simulink model "dVRK_RDOBS"  (Simulink 8.5)
settings: Solver=ode4  StartTime=0.0  StopTime=length(Tm)/1000  FixedStep=0.001  RelTol=1e-3
libraries: neural x630
(part 8 of 14)

== system dVRK_RDOBS/Joint 3 NN Dyn Ident/Layer 2/Delays 1 ==
  "p{2}" : Inport  PortDimensions=100  SampleTime=0.001
      mask Display: e = 0.06;c1 = [120 230 180]/255;c2 = ([120 230 180]+0)/(256+128);c3 = ([120 230 180]+128)/(256+128);patch([0 1 1 0],[0 0 1 1],c1);patch([0 1 1 1-e 1-e 0+e],[0 0 1 1-e 0+e 0+e],c2);patch([0 0 1 1-e 0+e 0+e],[0 1 1 1-e 1-e 0+e],c3);plot([0 1 1 0 0],[0 0 1 1 0]);
  mux : Mux  Inputs=1
      mask Display: e = 0.06;c1 = [120 150 230]/255;c2 = ([120 150 230]+0)/383;c3 = ([120 150 230]+128)/383;patch([0 1 1 0],[0 0 1 1],c1);patch([0 1 1 1-e 1-e 0+e],[0 0 1 1-e 0+e 0+e],c2);patch([0 0 1 1-e 0+e 0+e],[0 1 1 1-e 1-e 0+e],c3);plot([0 1 1 0 0],[0 0 1 1 0]);disp('Mux')
  "pd{2,1}" : Outport
      mask Display: e = 0.06;c1 = [120 230 180]/255;c2 = ([120 230 180]+0)/(256+128);c3 = ([120 230 180]+128)/(256+128);patch([0 1 1 0],[0 0 1 1],c1);patch([0 1 1 1-e 1-e 0+e],[0 0 1 1-e 0+e 0+e],c2);patch([0 0 1 1-e 0+e 0+e],[0 1 1 1-e 1-e 0+e],c3);plot([0 1 1 0 0],[0 0 1 1 0]);
  wires:
  "p{2}"/1 -> mux/1
  mux/1 -> "pd{2,1}"/1

== system dVRK_RDOBS/Joint 3 NN Dyn Ident/Layer 2/LW{2,1} ==
  "ad{2,1}" : Inport  PortDimensions=100  SampleTime=0.001
      mask Display: e = 0.06;c1 = [120 230 180]/255;c2 = ([120 230 180]+0)/(256+128);c3 = ([120 230 180]+128)/(256+128);patch([0 1 1 0],[0 0 1 1],c1);patch([0 1 1 1-e 1-e 0+e],[0 0 1 1-e 0+e 0+e],c2);patch([0 0 1 1-e 0+e 0+e],[0 1 1 1-e 1-e 0+e],c3);plot([0 1 1 0 0],[0 0 1 1 0]);
  "IW{2,1}(1,:)'" : Constant  Value=[-5.167254955505955;-1.8178436445965449;0.49211737404768147;-9.6830838662498326;-0.46755168693201082;1.7607856309859413;-0.084806969807460483;-1.5622860912871561;7.5100372282854364;-2.1948916538943264;0.1912546475987992;-3.4270018672278848;-7.3623865629808263;0.19766346350380701;0.48730997980870927;-0.20506493745529994;0.97745193864204638;0.16679036054209562;-0.17884970513459647;1.9736899383298294;-5.4772991886942579;-1.790933673981175;-3.5080464351406011;5.9822819492171488;2.8364180748438179;-0.2988913579922941;-0.072856020157372761;0.50318968999564839;2.3004396982929927;-0.15251543459787451;0.38654204560049144;-0.12940943559812457;2.832022145217802;-0.079145330621644708;-3.665648676122002;0.64287255965203383;3.931764786546037;-14.695817579739888;1.7362168126307793;0.36258126436183791;-1.9217057854420962;-0.29141146109069621;0.36160509862601681;0.76797790034887881;-1.7367991317149585;0.24018980699277243;-0.17825727249647286;-8.5366323143553746;0.13345769845967898;0.074840121060482059;1.4133773384275701;7.2423394399605971;0.070864353182638604;-0.10274757387060757;6.6363585532346834;0.60239026014106689;0.80956917570838027;0.62488754158380544;-0.17406692748002811;0.14812230476266114;-0.060128694573264654;0.56295323019274213;3.6621750916124358;-0.089541099264920349;-4.7357752009613723;0.19395813900816228;0.39853932795452873;0.14586909711395502;2.8018510438589299;-0.13038626499226821;0.50273892591220448;-0.17133267817527792;-0.22954196155175274;-0.54269745136298531;0.065188835392689465;-2.2926499451203948;0.3048007042901813;0.10233878512655985;0.42283871492618447;8.6505700551897551;-0.78592801250530531;12.737499354908245;0.47870971246031363;0.067869173127585336;0.14627490753962932;9.5380427871377513;0.32047634259962282;-0.056075778679940104;-0.09930934114651277;-0.5243064994596659;-0.12780387027723505;0.109605592652054;-0.87488691632775095;1.0204153757332541;0.13583268045024496;-4.9325290798337242;2.8671278081639411;-10.513906165852637;0.055350685358889748;-9.3050606724020604]
      mask Display: e = 0.06;c1 = [120 150 230]/255;c2 = ([120 150 230]+0)/383;c3 = ([120 150 230]+128)/383;patch([0 1 1 0],[0 0 1 1],c1);patch([0 1 1 1-e 1-e 0+e],[0 0 1 1-e 0+e 0+e],c2);patch([0 0 1 1-e 0+e 0+e],[0 1 1 1-e 1-e 0+e],c3);plot([0 1 1 0 0],[0 0 1 1 0]);disp('weights');
  Mux : Mux  Inputs=1
      mask Display: e = 0.06;c1 = [120 150 230]/255;c2 = ([120 150 230]+0)/383;c3 = ([120 150 230]+128)/383;patch([0 1 1 0],[0 0 1 1],c1);patch([0 1 1 1-e 1-e 0+e],[0 0 1 1-e 0+e 0+e],c2);patch([0 0 1 1-e 0+e 0+e],[0 1 1 1-e 1-e 0+e],c3);plot([0 1 1 0 0],[0 0 1 1 0]);disp('Mux');
  dotprod1 : neural/Weight Functions/dotprod
  "lz{2,1}" : Outport
      mask Display: e = 0.06;c1 = [120 230 180]/255;c2 = ([120 230 180]+0)/(256+128);c3 = ([120 230 180]+128)/(256+128);patch([0 1 1 0],[0 0 1 1],c1);patch([0 1 1 1-e 1-e 0+e],[0 0 1 1-e 0+e 0+e],c2);patch([0 0 1 1-e 0+e 0+e],[0 1 1 1-e 1-e 0+e],c3);plot([0 1 1 0 0],[0 0 1 1 0]);
  wires:
  "IW{2,1}(1,:)'"/1 -> dotprod1/1
  "ad{2,1}"/1 -> dotprod1/2
  dotprod1/1 -> Mux/1
  Mux/1 -> "lz{2,1}"/1

== system dVRK_RDOBS/Joint 4 NN Dyn Ident/Layer 1/Delays 1 ==
  "p{1}" : Inport  PortDimensions=12  SampleTime=0.001
      mask Display: e = 0.06;c1 = [120 230 180]/255;c2 = ([120 230 180]+0)/(256+128);c3 = ([120 230 180]+128)/(256+128);patch([0 1 1 0],[0 0 1 1],c1);patch([0 1 1 1-e 1-e 0+e],[0 0 1 1-e 0+e 0+e],c2);patch([0 0 1 1-e 0+e 0+e],[0 1 1 1-e 1-e 0+e],c3);plot([0 1 1 0 0],[0 0 1 1 0]);
  mux : Mux  Inputs=1
      mask Display: e = 0.06;c1 = [120 150 230]/255;c2 = ([120 150 230]+0)/383;c3 = ([120 150 230]+128)/383;patch([0 1 1 0],[0 0 1 1],c1);patch([0 1 1 1-e 1-e 0+e],[0 0 1 1-e 0+e 0+e],c2);patch([0 0 1 1-e 0+e 0+e],[0 1 1 1-e 1-e 0+e],c3);plot([0 1 1 0 0],[0 0 1 1 0]);disp('Mux')
  "pd{1,1}" : Outport
      mask Display: e = 0.06;c1 = [120 230 180]/255;c2 = ([120 230 180]+0)/(256+128);c3 = ([120 230 180]+128)/(256+128);patch([0 1 1 0],[0 0 1 1],c1);patch([0 1 1 1-e 1-e 0+e],[0 0 1 1-e 0+e 0+e],c2);patch([0 0 1 1-e 0+e 0+e],[0 1 1 1-e 1-e 0+e],c3);plot([0 1 1 0 0],[0 0 1 1 0]);
  wires:
  "p{1}"/1 -> mux/1
  mux/1 -> "pd{1,1}"/1
